simulink library "DYN_EPHEM"  (Simulink 10.1)
settings: Solver=VariableStepAuto  StartTime=0.0  StopTime=10.0  RelTol=1e-3
undefined symbols (not defined in the file): IAU, km, s
libraries: LIB_ROT x2, aerolibtransform2 x1, aerolibcelestial x1
settings Model: Creator=WilTravis  LastModifiedBy=m_mam

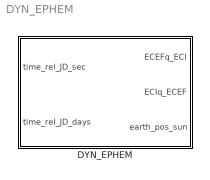
== system DYN_EPHEM ==
  DYN_EPHEM : Subsystem

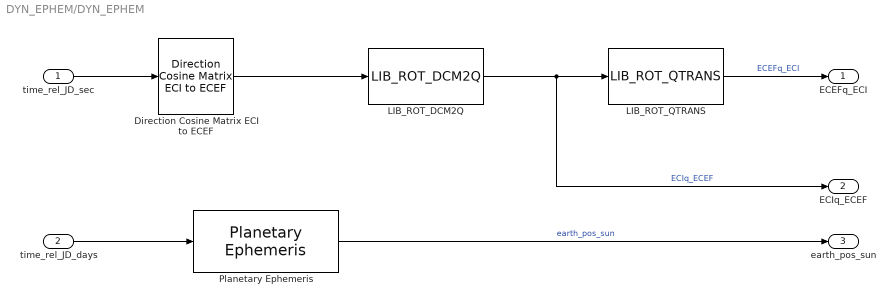
== system DYN_EPHEM/DYN_EPHEM ==
  "time_rel_JD_sec " : Inport
  time_rel_JD_days : Inport  Port=2
  Direction Cosine Matrix ECI to ECEF : aerolibtransform2/Direction Cosine Matrix ECI to ECEF  red=IAU-2000/2006  year=2018  month=January  day=1  hour=0  min=0  sec=0  deltaT=Sec  errorflag=None  extraparamflag=off
      settings: AttributesFormatString=%<red>  SourceProductBaseCode=AE
  LIB_ROT_DCM2Q : LIB_ROT/LIB_ROT_DCM2Q
  LIB_ROT_QTRANS : LIB_ROT/LIB_ROT_QTRANS
  Planetary Ephemeris : aerolibcelestial/Planetary Ephemeris  kmflag=km,km/s  epochflag=Julian date  de=DE405  nCenter=Sun  nTarget=Earth  errorflag=Error  velflag=off
      settings: AttributesFormatString=Ephemeris Data Unavailable  SourceProductBaseCode=AE
  ECEFq_ECI : Outport  VectorParamsAs1DForOutWhenUnconnected=off
  ECIq_ECEF : Outport  Port=2  VectorParamsAs1DForOutWhenUnconnected=off
  earth_pos_sun : Outport  Port=3  VectorParamsAs1DForOutWhenUnconnected=off
  wires:
  Planetary Ephemeris/1 -> earth_pos_sun/1  "earth_pos_sun"
  time_rel_JD_days/1 -> Planetary Ephemeris/1
  "time_rel_JD_sec "/1 -> Direction Cosine Matrix ECI to ECEF/1
  Direction Cosine Matrix ECI to ECEF/1 -> LIB_ROT_DCM2Q/1
  LIB_ROT_DCM2Q/1 -> ECIq_ECEF/1, LIB_ROT_QTRANS/1  "ECIq_ECEF"
  LIB_ROT_QTRANS/1 -> ECEFq_ECI/1  "ECEFq_ECI"
